simulink model "SF054A_PwrpkCmpbltyChk"  (R2013b)
settings: Solver=FixedStepDiscrete  SolverMode=SingleTasking  StartTime=0.0  StopTime=1  FixedStep=0.1  RelTol=1e-3
values from neighbouring files (symbols this model uses):
  CNVTOCNT_CNTPERMILLISEC_U32 = DataDict.Constant    [SF054A_PwrpkCmpbltyChk_DataDict.m]
  CORRLNFLTBIT2_CNT_U08 = DataDict.Constant    [SF054A_PwrpkCmpbltyChk_DataDict.m]
  CORRLNGEARIDFLTBIT3_CNT_U08 = DataDict.Constant    [SF054A_PwrpkCmpbltyChk_DataDict.m]
  GEARID1INVLBIT0_CNT_U08 = DataDict.Constant    [SF054A_PwrpkCmpbltyChk_DataDict.m]
  GEARID2INVLBIT1_CNT_U08 = DataDict.Constant    [SF054A_PwrpkCmpbltyChk_DataDict.m]
  NODEBSTEP_CNT_U16 = DataDict.Constant    [SF054A_PwrpkCmpbltyChk_DataDict.m]
  NOFAULT_CNT_U08 = DataDict.Constant    [SF054A_PwrpkCmpbltyChk_DataDict.m]
  PwrpkCmpbltyChkGearId = DataDict.Calibration    [SF054A_PwrpkCmpbltyChk_DataDict.m]
  TMRTHD_MILLISEC_U32 = DataDict.Constant    [SF054A_PwrpkCmpbltyChk_DataDict.m]
undefined symbols (not defined in the file or in its folder): NtcNr1, NtcSts1, SigQlfr1
libraries: simulink x10
(part 1 of 3)
settings Model: Creator=dzvc93  LastModifiedBy=DZVC93
settings SolverCC: AutoInsertRateTranBlk=on  InsertRTBMode=Always
settings DataIOCC: LimitDataPoints=off  SaveFormat=Structure  ReturnWorkspaceOutputs=on
settings OptimizationCC: BlockReduction=off  InlineParams=on  ZeroExternalMemoryAtStartup=off  ZeroInternalMemoryAtStartup=off  OptimizeModelRefInitCode=on  LifeSpan=1
settings DebuggingCC: SignalInfNanChecking=error  SignalRangeChecking=warning  UnderspecifiedInitializationDetection=Simplified  SolverPrmCheckMsg=error  InheritedTsInSrcMsg=error  DiscreteInheritContinuousMsg=error  SingleTaskRateTransMsg=error  TasksWithSamePriorityMsg=error  SigSpecEnsureSampleTimeMsg=error  CheckMatrixSingularityMsg=error  ParameterUnderflowMsg=error  ParameterPrecisionLossMsg=error  ParameterTunabilityLossMsg=error  FixptConstUnderflowMsg=warning  FixptConstOverflowMsg=warning  VectorMatrixConversionMsg=error  SignalLabelMismatchMsg=error  UnconnectedInputMsg=error  UnconnectedOutputMsg=error  UnconnectedLineMsg=error  SFcnCompatibilityMsg=error  UniqueDataStoreMsg=warning  BusObjectLabelMismatch=error  RootOutportRequireBusObject=error  AssertControl=DisableAll  ModelReferenceIOMsg=error  ModelReferenceVersionMismatchMessage=warning  ModelReferenceIOMismatchMessage=error  ModelReferenceCSMismatchMessage=warning  ModelReferenceDataLoggingMessage=error  StateNameClashWarn=warning  StrictBusMsg=ErrorOnBusTreatedAsVector  NonBusSignalsTreatedAsBus=error  SFUnexpectedBacktrackingDiag=error  SFInvalidInputDataAccessInChartInitDiag=error  SFNoUnconditionalDefaultTransitionDiag=error  SFTransitionOutsideNaturalParentDiag=error  SFUnconditionalTransitionShadowingDiag=error  SFUndirectedBroadcastEventsDiag=error
settings ModelReferenceCC: ModelReferenceNumInstancesAllowed=Single
settings RTWCC: SystemTargetFile=autosar.tlc  GenCodeOnly=on  TemplateMakefile=ert_default_tmf  Description=AUTOSAR  GenerateReport=on  ProcessScript=autosar_make_rtw_hook  LaunchReport=on
settings CodeAppCC: GenerateComments=off  IgnoreCustomStorageClasses=off  CustomSymbolStrType=$N$R$M  CustomSymbolStrBlkIO=$N$M  SimulinkBlockComments=off
settings STFCustomTargetCC: ParMdlRefBuildCompliant=on  CompOptLevelCompliant=on  IncludeMdlTerminateFcn=off  CombineOutputUpdateFcns=on  SuppressErrorStatus=on  ERTFirstTimeCompliant=on  ERTCustomFileBanners=on  SupportNonFinite=off  SupportComplex=off  SupportContinuousTime=off  SupportNonInlinedSFcns=off  MATLABClassNameForMDSCustomization=Simulink.SoftwareTarget.ERTCustomization  AutosarCompliant=on  GRTInterface=off  SystemTargetFile=autosar.tlc
settings ERTTargetCC: CodeReplacementLibrary=ANSI_C  ConcurrentExecutionCompliant=off  IncludeMdlTerminateFcn=off  SuppressErrorStatus=on  SupportNonFinite=off  SupportComplex=off  ModelStepFunctionPrototypeControlCompliant=off  CPPClassGenCompliant=off  AutosarCompliant=on  InlinedParameterPlacement=NonHierarchical  ERTCustomFileTemplate=example_file_process.tlc  EnableUserReplacementTypes=on

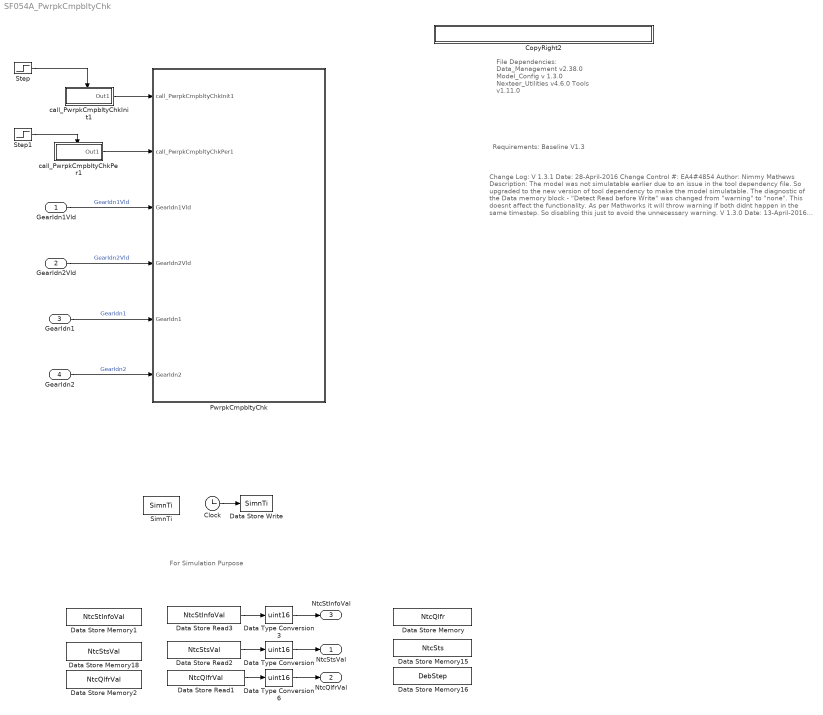
== system SF054A_PwrpkCmpbltyChk ==
  note: For Simulation Purpose
  note: Requirements: Baseline V1.3
  note: Change Log:
      |
      | V 1.3.1
      | Date: 28-April-2016
      | Change Control #: EA4#4854
      | Author: Nimmy Mathews
      | Description:
      | The model was not simulatable earlier due to an issue in the tool dependency file.
      | So upgraded to the new version of tool dependency to make the model simulatable.
      |
      | The diagnostic of the Data memory block - "Detect Read before Write" was changed
      | from "warning" to "none". This doesnt affect the functionality.
      | As per Mathworks it will throw warning if both didnt happen in the same timestep.
      | So disabling this just to avoid the unnecessary warning.
      |
      | V 1.3.0
      | Date: 13-April-2016
      | Change Control #: EA4#4854
      | Author: Nimmy Mathews
      | Description:
      | Typo error in GearId1Vld check where validation status should be changed
      | from false to true.
      | Traceability link to a different SF existed in the Fault block which was removed.
      |
      | V 1.2.0
      | Date: 11-April-2016
      | Change Control #: EA4#4854
      | Author: Nimmy Mathews
      | Description:
      | The NTC implementation changed to increase the throughput
      | The init function name changed to init1, changed both model and DD
      | false and true was introducted for fault status instead of 0 and 1
      |
      | V 1.1.0
      | Date: 6-April-2016
      | Change Control #: EA4#4854
      | Author: Nimmy Mathews
      | Description: Added NTC 1 Pager to SF054A FDD Package.
      |
      | V 1.0.0
      | Date: 28-March-2016
      | Change Control #: EA4#4854
      | Author: Nimmy Mathews
      | Description: Initial Baseline version of SF054A
  note: File Dependencies:
      |
      | Data_Management v2.38.0
      | Model_Config v 1.3.0
      | Nexteer_Utilities v4.6.0
      | Tools v1.11.0
  GearIdn1Vld : Inport
  GearIdn2Vld : Inport  Port=2
  GearIdn1 : Inport  Port=3
  GearIdn2 : Inport  Port=4  OutDataTypeStr=uint8
  Clock : Clock
  CopyRight2 : Subsystem  Description=|  mask(Copyright Information){none=on}
      | Copyright info block.                                               
      |                                                                     
      | Place copyright information at the top of every subsystem in design.
      mask prompts: none "No parameters"
      mask help: Place copyright information at the top of every subsystem in design.
      mask Display:
      | NxtrConf = 'Nexteer Confidential';
      | 
      | sys = bdroot; %handle for the current model ("system")
      | first = get_param(sys,'Created');
      | if(isempty(first))
      |     first = datestr(now,'yyyy');
      | else
      |     first = first(end-3:end);  %year is last four digits
      | end
      | 
      | last = get_param(sys,'LastModifiedDate');
      | if isempty(last)
      |     last = datestr(now,'yyyy');
      | else
      |     last = last(end-3:end);
      | end
      | 
      | if strcmp(first,last)
      |     fprintf('%s -- Copyright %s Nexteer',NxtrConf,first)
      | else
      |     fprintf('%s -- %s%s- %s Nexteer',NxtrConf,char(169),first,last)
      | end
  Data Store Memory : DataStoreMemory  DataStoreName=NtcQlfr  InitialValue=SigQlfr1.SIGQLFR_NORES  OutDataTypeStr=Enum: SigQlfr1
  Data Store Memory1 : DataStoreMemory  DataStoreName=NtcStInfoVal  OutDataTypeStr=uint8
  Data Store Memory15 : DataStoreMemory  DataStoreName=NtcSts  InitialValue=NtcSts1.NTCSTS_PREPASSD  OutDataTypeStr=Enum: NtcSts1
  Data Store Memory16 : DataStoreMemory  DataStoreName=DebStep
  Data Store Memory18 : DataStoreMemory  DataStoreName=NtcStsVal  InitialValue=NtcSts1.NTCSTS_PASSD  OutDataTypeStr=Enum: NtcSts1
  Data Store Memory2 : DataStoreMemory  DataStoreName=NtcQlfrVal  InitialValue=SigQlfr1.SIGQLFR_NORES  OutDataTypeStr=Enum: SigQlfr1
  Data Store Read1 : DataStoreRead  DataStoreName=NtcQlfrVal  SampleTime=0.1  DataStoreElements=NtcQlfrVal
  Data Store Read2 : DataStoreRead  DataStoreName=NtcStsVal  SampleTime=0.1  DataStoreElements=NtcStsVal
  Data Store Read3 : DataStoreRead  DataStoreName=NtcStInfoVal  SampleTime=0.1  DataStoreElements=NtcStInfoVal
  Data Store Write : DataStoreWrite  DataStoreName=SimnTi
  Data Type Conversion : DataTypeConversion  OutDataTypeStr=uint16
  Data Type Conversion3 : DataTypeConversion  OutDataTypeStr=uint16
  Data Type Conversion6 : DataTypeConversion  OutDataTypeStr=uint16
  PwrpkCmpbltyChk : Subsystem
  SimnTi : DataStoreMemory  DataStoreName=SimnTi
  Step : Step  Time=0.1  Before=1  After=0  SampleTime=0
  Step1 : Step  Time=0.1  SampleTime=0
  call_PwrpkCmpbltyChkInit1 : Subsystem  TreatAsAtomicUnit=on
  call_PwrpkCmpbltyChkPer1 : Subsystem  TreatAsAtomicUnit=on
  NtcStsVal : Outport
  NtcQlfrVal : Outport  Port=2
  NtcStInfoVal : Outport  Port=3
  wires:
  Clock/1 -> Data Store Write/1
  Data Type Conversion/1 -> NtcStsVal/1
  Data Store Read1/1 -> Data Type Conversion6/1
  Data Type Conversion6/1 -> NtcQlfrVal/1
  Data Store Read2/1 -> Data Type Conversion/1
  Data Type Conversion3/1 -> NtcStInfoVal/1
  Data Store Read3/1 -> Data Type Conversion3/1
  Step/1 -> call_PwrpkCmpbltyChkInit1/Enable
  Step1/1 -> call_PwrpkCmpbltyChkPer1/Enable
  call_PwrpkCmpbltyChkInit1/1(Out1) -> PwrpkCmpbltyChk/1(call_PwrpkCmpbltyChkInit1)
  call_PwrpkCmpbltyChkPer1/1(Out1) -> PwrpkCmpbltyChk/2(call_PwrpkCmpbltyChkPer1)
  GearIdn1Vld/1 -> PwrpkCmpbltyChk/3(GearIdn1Vld)  "GearIdn1Vld"
  GearIdn2/1 -> PwrpkCmpbltyChk/6(GearIdn2)  "GearIdn2"
  GearIdn2Vld/1 -> PwrpkCmpbltyChk/4(GearIdn2Vld)  "GearIdn2Vld"
  GearIdn1/1 -> PwrpkCmpbltyChk/5(GearIdn1)  "GearIdn1"

== system SF054A_PwrpkCmpbltyChk/CopyRight2 ==

== system SF054A_PwrpkCmpbltyChk/PwrpkCmpbltyChk ==
  note: SF054A            Powerpack Compatibility Check            Version: 1.3.1         Date: 28-April-2016
      |
      | This function verifies whether the Powerpack is compatible with the Gear. Appropriate failure messages shall be send based on the results of the compatibility check.
  call_PwrpkCmpbltyChkInit1 : Inport
  call_PwrpkCmpbltyChkPer1 : Inport  RequirementInfo="{'linktype_rmi_doors' '0000baba (/E-STEER Core/SubSystem Specifications/Application Functions/SF054A Powerpack Compatibility Check)' '#SF054A_43' 'true' 'REQ:  SF054A_43' '' } %GIDa_40f431f8_ed66_475b_95f6_ae44856e49ad"  Port=2
  GearIdn1Vld : Inport  RequirementInfo="{'linktype_rmi_doors' '0000baba (/E-STEER Core/SubSystem Specifications/Application Functions/SF054A Powerpack Compatibility Check)' '#SF054A_14' 'true' 'REQ:  SF054A_14' '' } %GIDa_5f31d6ee_7b00_4716_b73e_c3ac9d29cb03"  Port=3
  GearIdn2Vld : Inport  RequirementInfo="{'linktype_rmi_doors' '0000baba (/E-STEER Core/SubSystem Specifications/Application Functions/SF054A Powerpack Compatibility Check)' '#SF054A_60' 'true' 'REQ:  SF054A_60' '' } %GIDa_88de8345_4419_4889_8400_a234b2b9fc17"  Port=4
  GearIdn1 : Inport  RequirementInfo="{'linktype_rmi_doors' '0000baba (/E-STEER Core/SubSystem Specifications/Application Functions/SF054A Powerpack Compatibility Check)' '#SF054A_13' 'true' 'REQ:  SF054A_13' '' } %GIDa_d45d6377_e007_4fc8_a6ef_e1fd20e8e495"  Port=5
  GearIdn2 : Inport  RequirementInfo="{'linktype_rmi_doors' '0000baba (/E-STEER Core/SubSystem Specifications/Application Functions/SF054A Powerpack Compatibility Check)' '#SF054A_64' 'true' 'REQ:  SF054A_64' '' } %GIDa_6b853278_9304_4d85_aed7_bcabb0a88ac7"  Port=6
  CopyRight2 : Subsystem  Description=|  mask(Copyright Information){none=on}
      | Copyright info block.                                               
      |                                                                     
      | Place copyright information at the top of every subsystem in design.
      mask prompts: none "No parameters"
      mask help: Place copyright information at the top of every subsystem in design.
      mask Display:
      | NxtrConf = 'Nexteer Confidential';
      | 
      | sys = bdroot; %handle for the current model ("system")
      | first = get_param(sys,'Created');
      | if(isempty(first))
      |     first = datestr(now,'yyyy');
      | else
      |     first = first(end-3:end);  %year is last four digits
      | end
      | 
      | last = get_param(sys,'LastModifiedDate');
      | if isempty(last)
      |     last = datestr(now,'yyyy');
      | else
      |     last = last(end-3:end);
      | end
      | 
      | if strcmp(first,last)
      |     fprintf('%s -- Copyright %s Nexteer',NxtrConf,first)
      | else
      |     fprintf('%s -- %s%s- %s Nexteer',NxtrConf,char(169),first,last)
      | end
  Data Store Memory : DataStoreMemory  DataStoreName=GearIdnRefTmr  WriteAfterWriteMsg=warning  WriteAfterReadMsg=warning  StateMustResolveToSignalObject=on
  PwrpkCmpbltyChkInit1 : Subsystem  RequirementInfo="{'linktype_rmi_doors' '0000baba (/E-STEER Core/SubSystem Specifications/Application Functions/SF054A Powerpack Compatibility Check)' '#SF054A_80' 'true' 'REQ:  SF054A_80' '' ; 'linktype_rmi_doors' '0000baba (/E-STEER Core/SubSystem Specifications/Application Functions/SF054A Powerpack Compatibility Check)' '#SF054A_84' 'true' 'REQ:  SF054A_84' '' } %GIDa_5b0d0310_814e_45d4_b376_f8700ba71f1f"  TreatAsAtomicUnit=on
  PwrpkCmpbltyChkPer1 : Subsystem  TreatAsAtomicUnit=on
  wires:
  GearIdn1Vld/1 -> PwrpkCmpbltyChkPer1/1(GearIdn1Vld)
  GearIdn2/1 -> PwrpkCmpbltyChkPer1/4(GearIdn2)
  GearIdn2Vld/1 -> PwrpkCmpbltyChkPer1/2(GearIdn2Vld)
  GearIdn1/1 -> PwrpkCmpbltyChkPer1/3(GearIdn1)
  call_PwrpkCmpbltyChkInit1/1 -> PwrpkCmpbltyChkInit1/Trigger
  call_PwrpkCmpbltyChkPer1/1 -> PwrpkCmpbltyChkPer1/Trigger

== system SF054A_PwrpkCmpbltyChk/call_PwrpkCmpbltyChkInit1 ==
  Enable : EnablePort
  CopyRight2 : Subsystem  Description=|  mask(Copyright Information){none=on}
      | Copyright info block.                                               
      |                                                                     
      | Place copyright information at the top of every subsystem in design.
      mask prompts: none "No parameters"
      mask help: Place copyright information at the top of every subsystem in design.
      mask Display:
      | NxtrConf = 'Nexteer Confidential';
      | 
      | sys = bdroot; %handle for the current model ("system")
      | first = get_param(sys,'Created');
      | if(isempty(first))
      |     first = datestr(now,'yyyy');
      | else
      |     first = first(end-3:end);  %year is last four digits
      | end
      | 
      | last = get_param(sys,'LastModifiedDate');
      | if isempty(last)
      |     last = datestr(now,'yyyy');
      | else
      |     last = last(end-3:end);
      | end
      | 
      | if strcmp(first,last)
      |     fprintf('%s -- Copyright %s Nexteer',NxtrConf,first)
      | else
      |     fprintf('%s -- %s%s- %s Nexteer',NxtrConf,char(169),first,last)
      | end
  call_PwrpkCmpbltyChkInit1 : simulink/Ports & Subsystems/Function-Call Generator  sample_time=0.1  numberOfIterations=1
  Out1 : Outport
  wires:
  call_PwrpkCmpbltyChkInit1/1 -> Out1/1

== system SF054A_PwrpkCmpbltyChk/call_PwrpkCmpbltyChkPer1 ==
  Enable : EnablePort
  CopyRight2 : Subsystem  Description=|  mask(Copyright Information){none=on}
      | Copyright info block.                                               
      |                                                                     
      | Place copyright information at the top of every subsystem in design.
      mask prompts: none "No parameters"
      mask help: Place copyright information at the top of every subsystem in design.
      mask Display:
      | NxtrConf = 'Nexteer Confidential';
      | 
      | sys = bdroot; %handle for the current model ("system")
      | first = get_param(sys,'Created');
      | if(isempty(first))
      |     first = datestr(now,'yyyy');
      | else
      |     first = first(end-3:end);  %year is last four digits
      | end
      | 
      | last = get_param(sys,'LastModifiedDate');
      | if isempty(last)
      |     last = datestr(now,'yyyy');
      | else
      |     last = last(end-3:end);
      | end
      | 
      | if strcmp(first,last)
      |     fprintf('%s -- Copyright %s Nexteer',NxtrConf,first)
      | else
      |     fprintf('%s -- %s%s- %s Nexteer',NxtrConf,char(169),first,last)
      | end
  call_PwrpkCmpbltyChkPer1 : simulink/Ports & Subsystems/Function-Call Generator  RequirementInfo={} %GIDa_b9b5b09b_6cfc_4bbb_89a0_7902541bdf94  sample_time=0.1  numberOfIterations=1
  Out1 : Outport
  wires:
  call_PwrpkCmpbltyChkPer1/1 -> Out1/1

== system SF054A_PwrpkCmpbltyChk/PwrpkCmpbltyChk/CopyRight2 ==

== system SF054A_PwrpkCmpbltyChk/PwrpkCmpbltyChk/PwrpkCmpbltyChkInit1 ==
  note: Reference time is used to calculate the Elapsed time before which the Gear Id signals validity can be checked
  function : TriggerPort  TriggerType=function-call
  CopyRight2 : Subsystem  Description=|  mask(Copyright Information){none=on}
      | Copyright info block.                                               
      |                                                                     
      | Place copyright information at the top of every subsystem in design.
      mask prompts: none "No parameters"
      mask help: Place copyright information at the top of every subsystem in design.
      mask Display:
      | NxtrConf = 'Nexteer Confidential';
      | 
      | sys = bdroot; %handle for the current model ("system")
      | first = get_param(sys,'Created');
      | if(isempty(first))
      |     first = datestr(now,'yyyy');
      | else
      |     first = first(end-3:end);  %year is last four digits
      | end
      | 
      | last = get_param(sys,'LastModifiedDate');
      | if isempty(last)
      |     last = datestr(now,'yyyy');
      | else
      |     last = last(end-3:end);
      | end
      | 
      | if strcmp(first,last)
      |     fprintf('%s -- Copyright %s Nexteer',NxtrConf,first)
      | else
      |     fprintf('%s -- %s%s- %s Nexteer',NxtrConf,char(169),first,last)
      | end
  Data Store Write : DataStoreWrite  DataStoreName=GearIdnRefTmr
  GetRefTmr100MicroSec32bit : Subsystem
  wires:
  GetRefTmr100MicroSec32bit/1(RefTmr) -> Data Store Write/1

== system SF054A_PwrpkCmpbltyChk/PwrpkCmpbltyChk/PwrpkCmpbltyChkPer1 ==
  GearIdn1Vld : Inport
  GearIdn2Vld : Inport  Port=2
  GearIdn1 : Inport  Port=3
  GearIdn2 : Inport  Port=4
  function : TriggerPort  TriggerType=function-call
  CopyRight2 : Subsystem  Description=|  mask(Copyright Information){none=on}
      | Copyright info block.                                               
      |                                                                     
      | Place copyright information at the top of every subsystem in design.
      mask prompts: none "No parameters"
      mask help: Place copyright information at the top of every subsystem in design.
      mask Display:
      | NxtrConf = 'Nexteer Confidential';
      | 
      | sys = bdroot; %handle for the current model ("system")
      | first = get_param(sys,'Created');
      | if(isempty(first))
      |     first = datestr(now,'yyyy');
      | else
      |     first = first(end-3:end);  %year is last four digits
      | end
      | 
      | last = get_param(sys,'LastModifiedDate');
      | if isempty(last)
      |     last = datestr(now,'yyyy');
      | else
      |     last = last(end-3:end);
      | end
      | 
      | if strcmp(first,last)
      |     fprintf('%s -- Copyright %s Nexteer',NxtrConf,first)
      | else
      |     fprintf('%s -- %s%s- %s Nexteer',NxtrConf,char(169),first,last)
      | end
  Data Store Read : DataStoreRead  DataStoreName=GearIdnRefTmr
  FaultDetection : Subsystem  TreatAsAtomicUnit=on
  FaultHandling : Subsystem  TreatAsAtomicUnit=on
  wires:
  GearIdn2Vld/1 -> FaultDetection/3(GearIdn2Vld)
  GearIdn1Vld/1 -> FaultDetection/2(GearIdn1Vld)
  GearIdn1/1 -> FaultDetection/4(GearIdn1)
  GearIdn2/1 -> FaultDetection/5(GearIdn2)
  Data Store Read/1 -> FaultDetection/1(GearIdnRefTmr)  "GearIdnRefTmr"
  FaultDetection/8(GearIdCorrlnFltCnt) -> FaultHandling/8(GearIdCorrlnFltCnt)
  FaultDetection/7(CorrlnFltCnt) -> FaultHandling/7(CorrlnFltCnt)
  FaultDetection/6(GearIdn2FltCnt) -> FaultHandling/6(GearIdn2FltCnt)
  FaultDetection/5(GearIdn1FltCnt) -> FaultHandling/5(GearIdn1FltCnt)
  FaultDetection/4(GearIdCorrlnFltStat) -> FaultHandling/4(GearIdCorrlnFltStat)
  FaultDetection/3(CorrlnFltStat) -> FaultHandling/3(CorrlnFltStat)
  FaultDetection/1(GearIdn2FltStat) -> FaultHandling/1(GearIdn2FltStat)
  FaultDetection/2(GearIdn1FltStat) -> FaultHandling/2(GearIdn1FltStat)

== system SF054A_PwrpkCmpbltyChk/call_PwrpkCmpbltyChkInit1/CopyRight2 ==

== system SF054A_PwrpkCmpbltyChk/call_PwrpkCmpbltyChkPer1/CopyRight2 ==

== system SF054A_PwrpkCmpbltyChk/PwrpkCmpbltyChk/PwrpkCmpbltyChkInit1/CopyRight2 ==

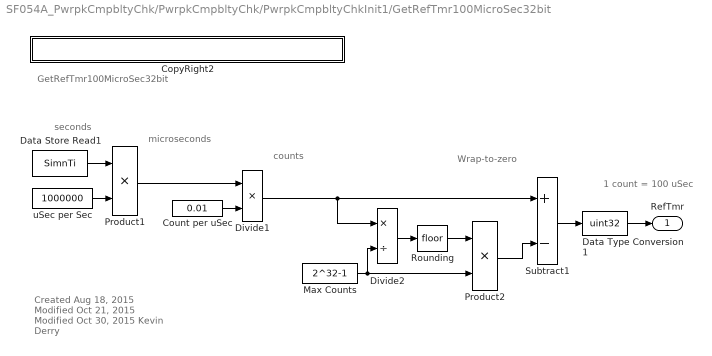
== system SF054A_PwrpkCmpbltyChk/PwrpkCmpbltyChk/PwrpkCmpbltyChkInit1/GetRefTmr100MicroSec32bit ==
  note: 1 count = 100 uSec
  note: seconds
  note: microseconds
  note: counts
  note: Wrap-to-zero
  note: GetRefTmr100MicroSec32bit
  note: Created Aug 18, 2015
      | Modified Oct 21, 2015
      | Modified Oct 30, 2015
      | Kevin Derry
  CopyRight2 : Subsystem  Description=|  mask(Copyright Information){none=on}
      | Copyright info block.                                               
      |                                                                     
      | Place copyright information at the top of every subsystem in design.
      mask prompts: none "No parameters"
      mask help: Place copyright information at the top of every subsystem in design.
      mask Display:
      | NxtrConf = 'Nexteer Confidential';
      | 
      | sys = bdroot; %handle for the current model ("system")
      | first = get_param(sys,'Created');
      | if(isempty(first))
      |     first = datestr(now,'yyyy');
      | else
      |     first = first(end-3:end);  %year is last four digits
      | end
      | 
      | last = get_param(sys,'LastModifiedDate');
      | if isempty(last)
      |     last = datestr(now,'yyyy');
      | else
      |     last = last(end-3:end);
      | end
      | 
      | if strcmp(first,last)
      |     fprintf('%s -- Copyright %s Nexteer',NxtrConf,first)
      | else
      |     fprintf('%s -- %s%s- %s Nexteer',NxtrConf,char(169),first,last)
      | end
  Count per uSec : Constant  Value=0.01
  Data Store Read1 : DataStoreRead  DataStoreName=SimnTi
  Data Type Conversion1 : DataTypeConversion  OutDataTypeStr=uint32
  Divide1 : Product  Inputs=**
  Divide2 : Product  Inputs=*/
  Max Counts : Constant  Value=2^32-1
  Product1 : Product
  Product2 : Product
  Rounding : Rounding
  Subtract1 : Sum  Inputs=+-
  uSec per Sec : Constant  Value=1000000
  RefTmr : Outport
  wires:
  Product2/1 -> Subtract1/2
  Subtract1/1 -> Data Type Conversion1/1
  Rounding/1 -> Product2/1
  Divide2/1 -> Rounding/1
  Max Counts/1 -> Divide2/2, Product2/2
  Divide1/1 -> Divide2/1, Subtract1/1
  Product1/1 -> Divide1/1
  Count per uSec/1 -> Divide1/2
  uSec per Sec/1 -> Product1/2
  Data Type Conversion1/1 -> RefTmr/1
  Data Store Read1/1 -> Product1/1

== system SF054A_PwrpkCmpbltyChk/PwrpkCmpbltyChk/PwrpkCmpbltyChkPer1/CopyRight2 ==

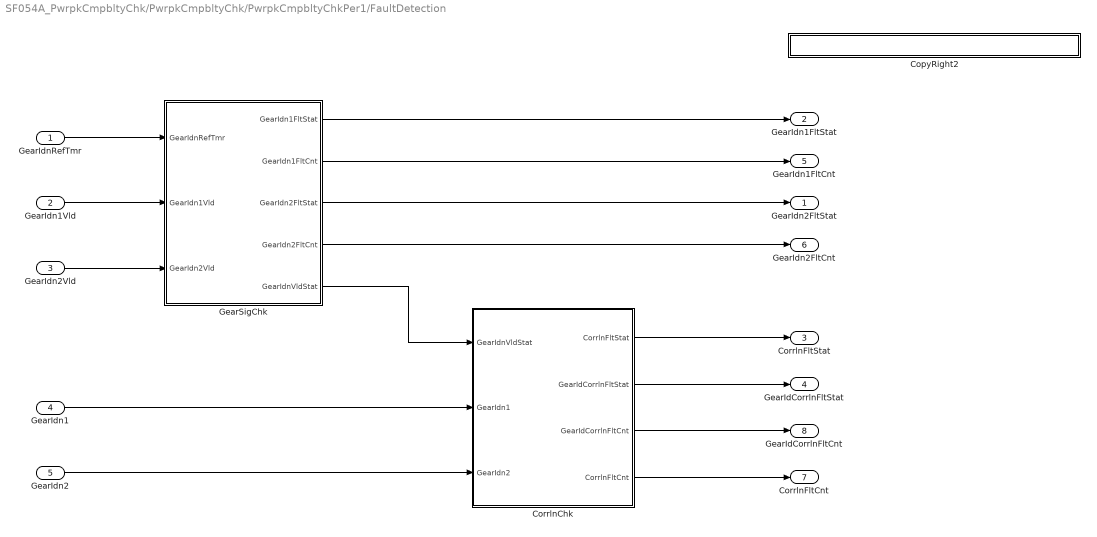
== system SF054A_PwrpkCmpbltyChk/PwrpkCmpbltyChk/PwrpkCmpbltyChkPer1/FaultDetection ==
  GearIdnRefTmr : Inport
  GearIdn1Vld : Inport  Port=2
  GearIdn2Vld : Inport  Port=3
  GearIdn1 : Inport  Port=4
  GearIdn2 : Inport  Port=5
  CopyRight2 : Subsystem  Description=|  mask(Copyright Information){none=on}
      | Copyright info block.                                               
      |                                                                     
      | Place copyright information at the top of every subsystem in design.
      mask prompts: none "No parameters"
      mask help: Place copyright information at the top of every subsystem in design.
      mask Display:
      | NxtrConf = 'Nexteer Confidential';
      | 
      | sys = bdroot; %handle for the current model ("system")
      | first = get_param(sys,'Created');
      | if(isempty(first))
      |     first = datestr(now,'yyyy');
      | else
      |     first = first(end-3:end);  %year is last four digits
      | end
      | 
      | last = get_param(sys,'LastModifiedDate');
      | if isempty(last)
      |     last = datestr(now,'yyyy');
      | else
      |     last = last(end-3:end);
      | end
      | 
      | if strcmp(first,last)
      |     fprintf('%s -- Copyright %s Nexteer',NxtrConf,first)
      | else
      |     fprintf('%s -- %s%s- %s Nexteer',NxtrConf,char(169),first,last)
      | end
  CorrlnChk : Subsystem  TreatAsAtomicUnit=on
  GearSigChk : Subsystem  RequirementInfo={} %GIDa_f2066328_55cd_431b_a5bf_6e7911fb5e96  TreatAsAtomicUnit=on
  GearIdn2FltStat : Outport
  GearIdn1FltStat : Outport  Port=2
  CorrlnFltStat : Outport  Port=3
  GearIdCorrlnFltStat : Outport  Port=4
  GearIdn1FltCnt : Outport  Port=5
  GearIdn2FltCnt : Outport  Port=6
  CorrlnFltCnt : Outport  Port=7
  GearIdCorrlnFltCnt : Outport  Port=8
  wires:
  GearIdn1Vld/1 -> GearSigChk/2(GearIdn1Vld)
  GearIdn2Vld/1 -> GearSigChk/3(GearIdn2Vld)
  CorrlnChk/2(GearIdCorrlnFltStat) -> GearIdCorrlnFltStat/1
  GearIdnRefTmr/1 -> GearSigChk/1(GearIdnRefTmr)
  GearIdn2/1 -> CorrlnChk/3(GearIdn2)
  GearIdn1/1 -> CorrlnChk/2(GearIdn1)
  CorrlnChk/3(GearIdCorrlnFltCnt) -> GearIdCorrlnFltCnt/1
  CorrlnChk/4(CorrlnFltCnt) -> CorrlnFltCnt/1
  GearSigChk/1(GearIdn1FltStat) -> GearIdn1FltStat/1
  CorrlnChk/1(CorrlnFltStat) -> CorrlnFltStat/1
  GearSigChk/5(GearIdnVldStat) -> CorrlnChk/1(GearIdnVldStat)
  GearSigChk/2(GearIdn1FltCnt) -> GearIdn1FltCnt/1
  GearSigChk/3(GearIdn2FltStat) -> GearIdn2FltStat/1
  GearSigChk/4(GearIdn2FltCnt) -> GearIdn2FltCnt/1

== system SF054A_PwrpkCmpbltyChk/PwrpkCmpbltyChk/PwrpkCmpbltyChkPer1/FaultHandling ==
  GearIdn2FltStat : Inport
  GearIdn1FltStat : Inport  Port=2
  CorrlnFltStat : Inport  Port=3
  GearIdCorrlnFltStat : Inport  Port=4
  GearIdn1FltCnt : Inport  Port=5
  GearIdn2FltCnt : Inport  Port=6
  CorrlnFltCnt : Inport  Port=7
  GearIdCorrlnFltCnt : Inport  Port=8
  CopyRight2 : Subsystem  Description=|  mask(Copyright Information){none=on}
      | Copyright info block.                                               
      |                                                                     
      | Place copyright information at the top of every subsystem in design.
      mask prompts: none "No parameters"
      mask help: Place copyright information at the top of every subsystem in design.
      mask Display:
      | NxtrConf = 'Nexteer Confidential';
      | 
      | sys = bdroot; %handle for the current model ("system")
      | first = get_param(sys,'Created');
      | if(isempty(first))
      |     first = datestr(now,'yyyy');
      | else
      |     first = first(end-3:end);  %year is last four digits
      | end
      | 
      | last = get_param(sys,'LastModifiedDate');
      | if isempty(last)
      |     last = datestr(now,'yyyy');
      | else
      |     last = last(end-3:end);
      | end
      | 
      | if strcmp(first,last)
      |     fprintf('%s -- Copyright %s Nexteer',NxtrConf,first)
      | else
      |     fprintf('%s -- %s%s- %s Nexteer',NxtrConf,char(169),first,last)
      | end
  FaultSelection : Subsystem  RequirementInfo="{'linktype_rmi_doors' '0000baba (/E-STEER Core/SubSystem Specifications/Application Functions/SF054A Powerpack Compatibility Check)' '#SF054A_93' 'true' 'REQ:  SF054A_93' '' ; 'linktype_rmi_doors' '0000baba (/E-STEER Core/SubSystem Specifications/Application Functions/SF054A Powerpack Compatibility Check)' '#SF054A_97' 'true' 'REQ:  SF054A_97' '' ; 'linktype_rmi_doors' '0000baba (/E-STEER Core/SubSystem Specifications/Application Functions/SF054A Powerpack Compatibility Check)' '#SF054A_94' 'true' 'REQ:  SF054A_94' '' ; 'linktype_rmi_doors' '0000baba (/E-STEER Core/SubSystem Specifications/Application Functions/SF054A Powerpack Compatibility Check)' '#SF054A_95' 'true' 'REQ:  SF054A_95' '' ; 'linktype_rmi_doors' '0000baba (/E-STEER Core/SubSystem Specifications/Application Functions/SF054A Powerpack Compatibility Check)' '#SF054A_96' 'true' 'REQ:  SF054A_96' '' } %GIDa_16b1e10d_add9_4ba3_9e5d_552278990ffe"  TreatAsAtomicUnit=on
  NTC : Subsystem  Priority=2  TreatAsAtomicUnit=on
  NTCCheck : Subsystem
  wires:
  GearIdn2FltCnt/1 -> FaultSelection/6(GearIdn2FltCnt)
  GearIdn2FltStat/1 -> FaultSelection/1(GearIdn2FltStat)
  GearIdCorrlnFltCnt/1 -> FaultSelection/8(GearIdCorrlnFltCnt)
  CorrlnFltStat/1 -> FaultSelection/3(CorrlnFltStat)
  GearIdn1FltCnt/1 -> FaultSelection/5(GearIdn1FltCnt)
  CorrlnFltCnt/1 -> FaultSelection/7(CorrlnFltCnt)
  GearIdn1FltStat/1 -> FaultSelection/2(GearIdn1FltStat)
  GearIdCorrlnFltStat/1 -> FaultSelection/4(GearIdCorrlnFltStat)
  FaultSelection/1(FltStat) -> NTC/1(FltStat), NTCCheck/1(FltStat)
  NTCCheck/1(NTC_Condition) -> NTC/Action
  FaultSelection/2(FLT_CNT_U08) -> NTC/2(FLT_CNT_U08)

== system SF054A_PwrpkCmpbltyChk/PwrpkCmpbltyChk/PwrpkCmpbltyChkInit1/GetRefTmr100MicroSec32bit/CopyRight2 ==

== system SF054A_PwrpkCmpbltyChk/PwrpkCmpbltyChk/PwrpkCmpbltyChkPer1/FaultDetection/CopyRight2 ==

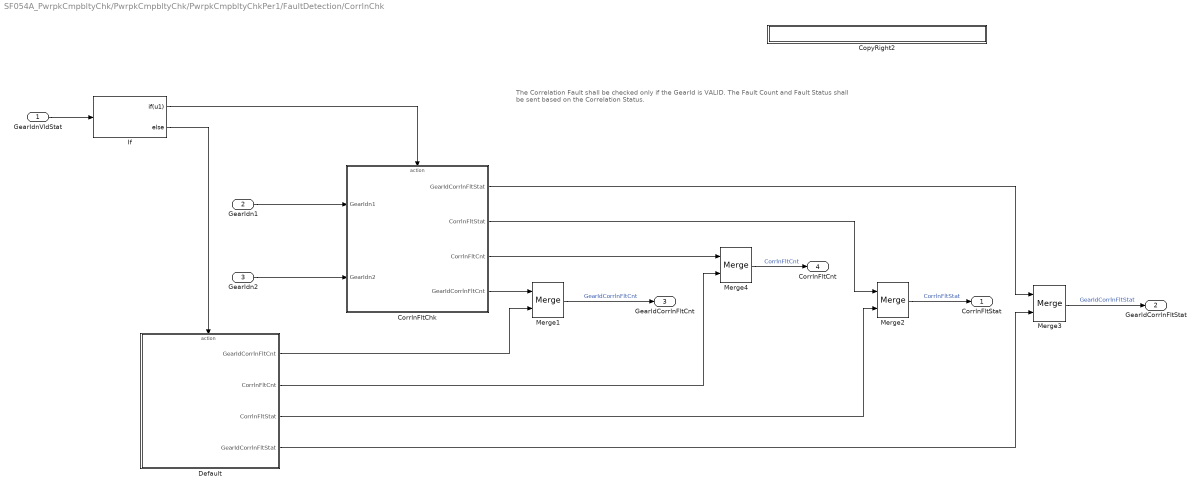
== system SF054A_PwrpkCmpbltyChk/PwrpkCmpbltyChk/PwrpkCmpbltyChkPer1/FaultDetection/CorrlnChk ==
  note: The Correlation Fault shall be checked only if the GearId is VALID.
      | The Fault Count and Fault Status shall be sent based on the Correlation Status.
  GearIdnVldStat : Inport
  GearIdn1 : Inport  Port=2
  GearIdn2 : Inport  Port=3
  CopyRight2 : Subsystem  Description=|  mask(Copyright Information){none=on}
      | Copyright info block.                                               
      |                                                                     
      | Place copyright information at the top of every subsystem in design.
      mask prompts: none "No parameters"
      mask help: Place copyright information at the top of every subsystem in design.
      mask Display:
      | NxtrConf = 'Nexteer Confidential';
      | 
      | sys = bdroot; %handle for the current model ("system")
      | first = get_param(sys,'Created');
      | if(isempty(first))
      |     first = datestr(now,'yyyy');
      | else
      |     first = first(end-3:end);  %year is last four digits
      | end
      | 
      | last = get_param(sys,'LastModifiedDate');
      | if isempty(last)
      |     last = datestr(now,'yyyy');
      | else
      |     last = last(end-3:end);
      | end
      | 
      | if strcmp(first,last)
      |     fprintf('%s -- Copyright %s Nexteer',NxtrConf,first)
      | else
      |     fprintf('%s -- %s%s- %s Nexteer',NxtrConf,char(169),first,last)
      | end
  CorrlnFltChk : Subsystem  TreatAsAtomicUnit=on
  Default : Subsystem  RequirementInfo="{'linktype_rmi_doors' '0000baba (/E-STEER Core/SubSystem Specifications/Application Functions/SF054A Powerpack Compatibility Check)' '#SF054A_67' 'true' 'REQ:  SF054A_67' '' } %GIDa_def38050_3538_46ff_9893_cae5c22fdef7"  TreatAsAtomicUnit=on
  If : If  RequirementInfo="{'linktype_rmi_doors' '0000ba59 (/E-STEER Core/SubSystem Specifications/Application Functions/SF011A Learned EOT Limits)' '#SF011A_128' 'true' 'REQ:  SF011A_128' '' ; 'linktype_rmi_doors' '0000ba59 (/E-STEER Core/SubSystem Specifications/Application Functions/SF011A Learned EOT Limits)' '#SF011A_143' 'true' 'REQ:  SF011A_143' '' ; 'linktype_rmi_doors' '0000baba (/E-STEER Core/SubSystem Specifications/Application Functions/SF054A Powerpack Compatibility Check)' '#SF054A_92' 'true' 'REQ:  SF054A_92' '' } %GIDa_88644833_66a6_4b0c_a623_ac53310b9524"  Priority=0  IfExpression=u1
  Merge{1..4} (4 alike) : Merge
  CorrlnFltStat : Outport
  GearIdCorrlnFltStat : Outport  Port=2
  GearIdCorrlnFltCnt : Outport  Port=3
  CorrlnFltCnt : Outport  Port=4
  wires:
  If/1 -> CorrlnFltChk/Action
  GearIdnVldStat/1 -> If/1
  If/2 -> Default/Action
  GearIdn1/1 -> CorrlnFltChk/1(GearIdn1)
  GearIdn2/1 -> CorrlnFltChk/2(GearIdn2)
  CorrlnFltChk/4(GearIdCorrlnFltCnt) -> Merge1/1
  Default/1(GearIdCorrlnFltCnt) -> Merge1/2
  CorrlnFltChk/3(CorrlnFltCnt) -> Merge4/1
  Default/2(CorrlnFltCnt) -> Merge4/2
  Merge4/1 -> CorrlnFltCnt/1  "CorrlnFltCnt"
  Merge1/1 -> GearIdCorrlnFltCnt/1  "GearIdCorrlnFltCnt"
  CorrlnFltChk/2(CorrlnFltStat) -> Merge2/1
  Default/3(CorrlnFltStat) -> Merge2/2
  Merge2/1 -> CorrlnFltStat/1  "CorrlnFltStat"
  Default/4(GearIdCorrlnFltStat) -> Merge3/2
  CorrlnFltChk/1(GearIdCorrlnFltStat) -> Merge3/1
  Merge3/1 -> GearIdCorrlnFltStat/1  "GearIdCorrlnFltStat"

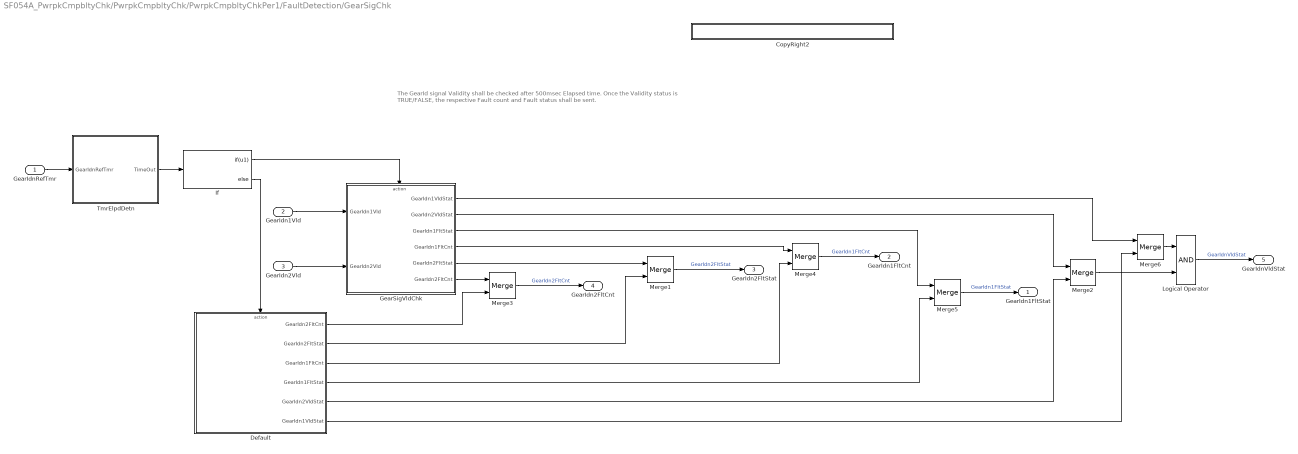
== system SF054A_PwrpkCmpbltyChk/PwrpkCmpbltyChk/PwrpkCmpbltyChkPer1/FaultDetection/GearSigChk ==
  note: The GearId signal Validity shall be checked after 500msec Elapsed time.
      | Once the Validity status is TRUE/FALSE, the respective Fault count and Fault status shall be sent.
  GearIdnRefTmr : Inport
  GearIdn1Vld : Inport  RequirementInfo="{'linktype_rmi_doors' '0000baba (/E-STEER Core/SubSystem Specifications/Application Functions/SF054A Powerpack Compatibility Check)' '#SF054A_13' 'true' 'REQ:  SF054A_13' '' } %GIDa_07141503_f391_43d0_b4ae_981cf6a36717"  Port=2
  GearIdn2Vld : Inport  RequirementInfo="{'linktype_rmi_doors' '0000baba (/E-STEER Core/SubSystem Specifications/Application Functions/SF054A Powerpack Compatibility Check)' '#SF054A_64' 'true' 'REQ:  SF054A_64' '' } %GIDa_7408e6e2_7c0d_4759_ac65_8b3622c7b954"  Port=3
  CopyRight2 : Subsystem  Description=|  mask(Copyright Information){none=on}
      | Copyright info block.                                               
      |                                                                     
      | Place copyright information at the top of every subsystem in design.
      mask prompts: none "No parameters"
      mask help: Place copyright information at the top of every subsystem in design.
      mask Display:
      | NxtrConf = 'Nexteer Confidential';
      | 
      | sys = bdroot; %handle for the current model ("system")
      | first = get_param(sys,'Created');
      | if(isempty(first))
      |     first = datestr(now,'yyyy');
      | else
      |     first = first(end-3:end);  %year is last four digits
      | end
      | 
      | last = get_param(sys,'LastModifiedDate');
      | if isempty(last)
      |     last = datestr(now,'yyyy');
      | else
      |     last = last(end-3:end);
      | end
      | 
      | if strcmp(first,last)
      |     fprintf('%s -- Copyright %s Nexteer',NxtrConf,first)
      | else
      |     fprintf('%s -- %s%s- %s Nexteer',NxtrConf,char(169),first,last)
      | end
  Default : Subsystem  RequirementInfo="{'linktype_rmi_doors' '0000baba (/E-STEER Core/SubSystem Specifications/Application Functions/SF054A Powerpack Compatibility Check)' '#SF054A_80' 'true' 'REQ:  SF054A_80' '' ; 'linktype_rmi_doors' '0000baba (/E-STEER Core/SubSystem Specifications/Application Functions/SF054A Powerpack Compatibility Check)' '#SF054A_84' 'true' 'REQ:  SF054A_84' '' } %GIDa_7f3eb837_d03b_4751_b310_4fff8ae8046f"  TreatAsAtomicUnit=on
  GearSigVldChk : Subsystem  RequirementInfo="{'linktype_rmi_doors' '0000baba (/E-STEER Core/SubSystem Specifications/Application Functions/SF054A Powerpack Compatibility Check)' '#SF054A_80' 'true' 'REQ:  SF054A_80' '' ; 'linktype_rmi_doors' '0000baba (/E-STEER Core/SubSystem Specifications/Application Functions/SF054A Powerpack Compatibility Check)' '#SF054A_84' 'true' 'REQ:  SF054A_84' '' } %GIDa_50918e26_72db_460e_87dd_1d09ff0e4a92"  TreatAsAtomicUnit=on
  If : If  RequirementInfo="{'linktype_rmi_doors' '0000ba59 (/E-STEER Core/SubSystem Specifications/Application Functions/SF011A Learned EOT Limits)' '#SF011A_128' 'true' 'REQ:  SF011A_128' '' ; 'linktype_rmi_doors' '0000ba59 (/E-STEER Core/SubSystem Specifications/Application Functions/SF011A Learned EOT Limits)' '#SF011A_143' 'true' 'REQ:  SF011A_143' '' } %GIDa_cd94ec7e_13a5_465e_9cb0_d9971a6d12eb"  Priority=0  IfExpression=u1
  Logical Operator : Logic  RequirementInfo="{'linktype_rmi_doors' '0000baba (/E-STEER Core/SubSystem Specifications/Application Functions/SF054A Powerpack Compatibility Check)' '#SF054A_92' 'true' 'REQ:  SF054A_92' '' } %GIDa_5e2c5032_9bae_408f_9cc9_2f404b5ee79c"  AllPortsSameDT=off  OutDataTypeStr=boolean
  Merge1 : Merge  RequirementInfo="{'linktype_rmi_doors' '0000baba (/E-STEER Core/SubSystem Specifications/Application Functions/SF054A Powerpack Compatibility Check)' '#SF054A_84' 'true' 'REQ:  SF054A_84' '' } %GIDa_bec317ef_b7a4_4614_b9ad_28b5a9025cda"
  Merge2 : Merge  RequirementInfo="{'linktype_rmi_doors' '0000baba (/E-STEER Core/SubSystem Specifications/Application Functions/SF054A Powerpack Compatibility Check)' '#SF054A_84' 'true' 'REQ:  SF054A_84' '' } %GIDa_6bc901bf_c68c_4fb5_a62e_c8ea77f1fe85"
  Merge3 : Merge  RequirementInfo="{'linktype_rmi_doors' '0000baba (/E-STEER Core/SubSystem Specifications/Application Functions/SF054A Powerpack Compatibility Check)' '#SF054A_84' 'true' 'REQ:  SF054A_84' '' } %GIDa_e9fdb361_5db9_41db_8825_56448b17746d"
  Merge4 : Merge  RequirementInfo="{'linktype_rmi_doors' '0000baba (/E-STEER Core/SubSystem Specifications/Application Functions/SF054A Powerpack Compatibility Check)' '#SF054A_84' 'true' 'REQ:  SF054A_84' '' } %GIDa_e78dec43_3536_4a72_9dfe_8afa78627e64"
  Merge5 : Merge  RequirementInfo="{'linktype_rmi_doors' '0000baba (/E-STEER Core/SubSystem Specifications/Application Functions/SF054A Powerpack Compatibility Check)' '#SF054A_80' 'true' 'REQ:  SF054A_80' '' } %GIDa_1eff8661_cf07_4a78_8db4_5b8c4cf59720"
  Merge6 : Merge  RequirementInfo="{'linktype_rmi_doors' '0000baba (/E-STEER Core/SubSystem Specifications/Application Functions/SF054A Powerpack Compatibility Check)' '#SF054A_84' 'true' 'REQ:  SF054A_84' '' } %GIDa_8b70efac_3bbf_4a8d_9aad_8acce263dfb5"
  TmrElpdDetn : Subsystem  RequirementInfo="{'linktype_rmi_doors' '0000baba (/E-STEER Core/SubSystem Specifications/Application Functions/SF054A Powerpack Compatibility Check)' '#SF054A_80' 'true' 'REQ:  SF054A_80' '' ; 'linktype_rmi_doors' '0000baba (/E-STEER Core/SubSystem Specifications/Application Functions/SF054A Powerpack Compatibility Check)' '#SF054A_84' 'true' 'REQ:  SF054A_84' '' } %GIDa_3d8132f7_1416_4119_8569_27da00ff5b04"  TreatAsAtomicUnit=on
  GearIdn1FltStat : Outport  RequirementInfo="{'linktype_rmi_doors' '0000baba (/E-STEER Core/SubSystem Specifications/Application Functions/SF054A Powerpack Compatibility Check)' '#SF054A_84' 'true' 'REQ:  SF054A_84' '' } %GIDa_b46c068e_ca4a_4d3a_af26_9ece79e7d35d"
  GearIdn1FltCnt : Outport  RequirementInfo="{'linktype_rmi_doors' '0000baba (/E-STEER Core/SubSystem Specifications/Application Functions/SF054A Powerpack Compatibility Check)' '#SF054A_84' 'true' 'REQ:  SF054A_84' '' } %GIDa_7f5e250d_fa59_4e89_bb25_1e9b18886f22"  Port=2
  GearIdn2FltStat : Outport  RequirementInfo="{'linktype_rmi_doors' '0000baba (/E-STEER Core/SubSystem Specifications/Application Functions/SF054A Powerpack Compatibility Check)' '#SF054A_84' 'true' 'REQ:  SF054A_84' '' } %GIDa_66dbd4fe_ddce_4353_aa0a_56a3a23deafb"  Port=3
  GearIdn2FltCnt : Outport  RequirementInfo="{'linktype_rmi_doors' '0000baba (/E-STEER Core/SubSystem Specifications/Application Functions/SF054A Powerpack Compatibility Check)' '#SF054A_84' 'true' 'REQ:  SF054A_84' '' } %GIDa_7cf17f66_febb_4ac9_8969_995d7f8842e9"  Port=4
  GearIdnVldStat : Outport  RequirementInfo="{'linktype_rmi_doors' '0000baba (/E-STEER Core/SubSystem Specifications/Application Functions/SF054A Powerpack Compatibility Check)' '#SF054A_92' 'true' 'REQ:  SF054A_92' '' } %GIDa_d7988670_a7e1_4d5f_84ff_78bb6246dbb5"  Port=5
  wires:
  GearIdn2Vld/1 -> GearSigVldChk/2(GearIdn2Vld)
  GearIdn1Vld/1 -> GearSigVldChk/1(GearIdn1Vld)
  GearIdnRefTmr/1 -> TmrElpdDetn/1(GearIdnRefTmr)
  TmrElpdDetn/1(TimeOut) -> If/1
  If/1 -> GearSigVldChk/Action
  If/2 -> Default/Action
  Logical Operator/1 -> GearIdnVldStat/1  "GearIdnVldStat"
  Merge2/1 -> Logical Operator/2
  GearSigVldChk/6(GearIdn2FltCnt) -> Merge3/1
  Default/1(GearIdn2FltCnt) -> Merge3/2
  Merge3/1 -> GearIdn2FltCnt/1  "GearIdn2FltCnt"
  Default/2(GearIdn2FltStat) -> Merge1/2
  GearSigVldChk/5(GearIdn2FltStat) -> Merge1/1
  Merge1/1 -> GearIdn2FltStat/1  "GearIdn2FltStat"
  Merge4/1 -> GearIdn1FltCnt/1  "GearIdn1FltCnt"
  Merge5/1 -> GearIdn1FltStat/1  "GearIdn1FltStat"
  GearSigVldChk/4(GearIdn1FltCnt) -> Merge4/1
  Default/3(GearIdn1FltCnt) -> Merge4/2
  Default/4(GearIdn1FltStat) -> Merge5/2
  GearSigVldChk/3(GearIdn1FltStat) -> Merge5/1
  GearSigVldChk/2(GearIdn2VldStat) -> Merge2/1
  Default/5(GearIdn2VldStat) -> Merge2/2
  GearSigVldChk/1(GearIdn1VldStat) -> Merge6/1
  Default/6(GearIdn1VldStat) -> Merge6/2
  Merge6/1 -> Logical Operator/1

== system SF054A_PwrpkCmpbltyChk/PwrpkCmpbltyChk/PwrpkCmpbltyChkPer1/FaultHandling/CopyRight2 ==

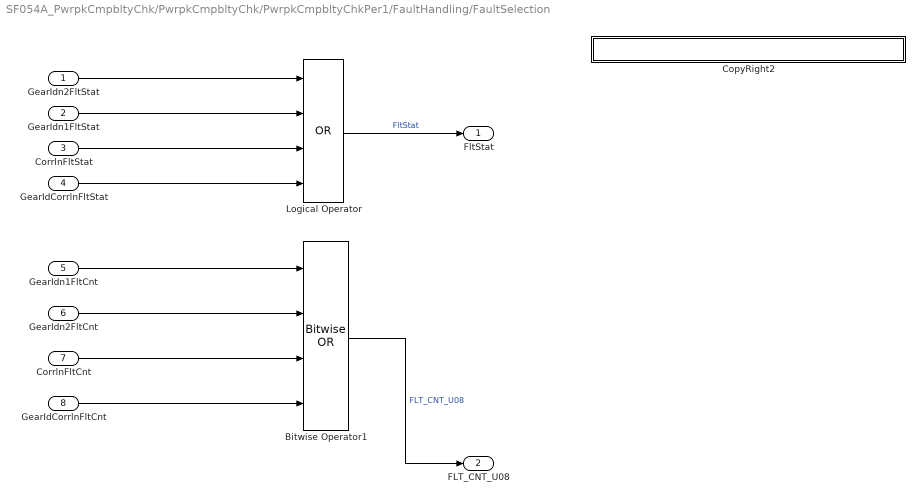
== system SF054A_PwrpkCmpbltyChk/PwrpkCmpbltyChk/PwrpkCmpbltyChkPer1/FaultHandling/FaultSelection ==
  GearIdn2FltStat : Inport
  GearIdn1FltStat : Inport  Port=2
  CorrlnFltStat : Inport  Port=3
  GearIdCorrlnFltStat : Inport  Port=4
  GearIdn1FltCnt : Inport  Port=5
  GearIdn2FltCnt : Inport  Port=6
  CorrlnFltCnt : Inport  Port=7
  GearIdCorrlnFltCnt : Inport  Port=8
  Bitwise Operator1 : simulink/Logic and Bit Operations/Bitwise Operator  logicop=OR  UseBitMask=off  NumInputPorts=4  BitMask=bin2dec('11011001')  BitMaskRealWorld=Stored Integer
  CopyRight2 : Subsystem  Description=|  mask(Copyright Information){none=on}
      | Copyright info block.                                               
      |                                                                     
      | Place copyright information at the top of every subsystem in design.
      mask prompts: none "No parameters"
      mask help: Place copyright information at the top of every subsystem in design.
      mask Display:
      | NxtrConf = 'Nexteer Confidential';
      | 
      | sys = bdroot; %handle for the current model ("system")
      | first = get_param(sys,'Created');
      | if(isempty(first))
      |     first = datestr(now,'yyyy');
      | else
      |     first = first(end-3:end);  %year is last four digits
      | end
      | 
      | last = get_param(sys,'LastModifiedDate');
      | if isempty(last)
      |     last = datestr(now,'yyyy');
      | else
      |     last = last(end-3:end);
      | end
      | 
      | if strcmp(first,last)
      |     fprintf('%s -- Copyright %s Nexteer',NxtrConf,first)
      | else
      |     fprintf('%s -- %s%s- %s Nexteer',NxtrConf,char(169),first,last)
      | end
  Logical Operator : Logic  Operator=OR  Inputs=4  AllPortsSameDT=off  OutDataTypeStr=boolean
  FltStat : Outport
  FLT_CNT_U08 : Outport  Port=2
  wires:
  GearIdn2FltStat/1 -> Logical Operator/1
  GearIdCorrlnFltStat/1 -> Logical Operator/4
  GearIdn1FltStat/1 -> Logical Operator/2
  CorrlnFltStat/1 -> Logical Operator/3
  Bitwise Operator1/1 -> FLT_CNT_U08/1  "FLT_CNT_U08"
  GearIdn1FltCnt/1 -> Bitwise Operator1/1
  GearIdn2FltCnt/1 -> Bitwise Operator1/2
  CorrlnFltCnt/1 -> Bitwise Operator1/3
  GearIdCorrlnFltCnt/1 -> Bitwise Operator1/4
  Logical Operator/1 -> FltStat/1  "FltStat"
